simulink model "change_watcher"  (R2021a)
settings: configuration reference "f2_ctrl_config" (kept outside this file)
libraries: simulink x2
settings Model: DataDictionary=motor_data.sldd  EnableAccessToBaseWorkspace=off  Creator=Litao  LastModifiedBy=Litao
settings ConfigSetRef: SourceName=f2_ctrl_config

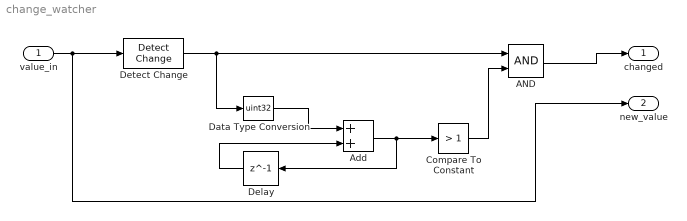
== system change_watcher ==
  value_in : Inport  OutDataTypeStr=int16
  AND : Logic  AllPortsSameDT=off  OutDataTypeStr=boolean
  Add : Sum
  Compare To Constant : simulink/Logic and Bit Operations/Compare To Constant  relop=>  const=1  OutDataTypeStr=boolean
  Data Type Conversion : DataTypeConversion  OutDataTypeStr=uint32
  Delay : Delay  DelayLength=1  InitialCondition=0
  Detect Change : simulink/Logic and Bit Operations/Detect Change  vinit=0  OutDataTypeStr=boolean
  changed : Outport
  new_value : Outport  Port=2
  wires:
  Detect Change/1 -> Data Type Conversion/1, AND/1
  AND/1 -> changed/1
  Add/1 -> Compare To Constant/1, Delay/1
  Delay/1 -> Add/2
  Data Type Conversion/1 -> Add/1
  Compare To Constant/1 -> AND/2
  value_in/1 -> new_value/1, Detect Change/1
